simulink model "Simulink_AM"  (R2020b)
settings: Solver=VariableStepAuto  StartTime=0.0  StopTime=10.0  RelTol=1e-3
libraries: dsparch4 x2
settings Model: Creator=enrique  LastModifiedBy=enrique

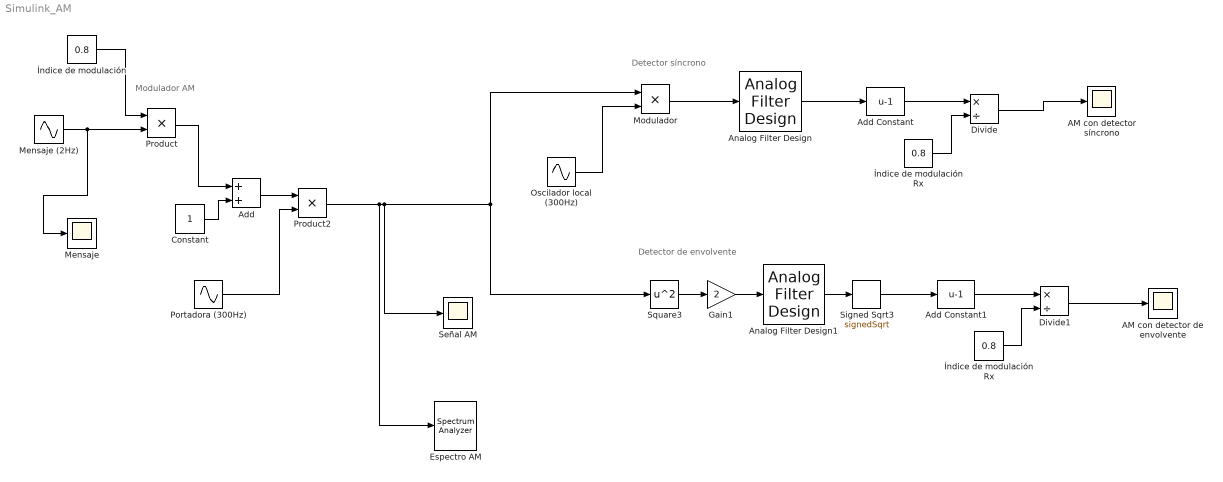
== system Simulink_AM ==
  note: Detector de envolvente
  note: Detector síncrono
  note: Modulador AM
  AM con detector de envolvente : Scope
  AM con detector síncrono : Scope
  Add : Sum
  Add Constant : Bias  Bias=-1
  Add Constant1 : Bias  Bias=-1
  Analog Filter Design : dsparch4/Analog Filter Design  method=Butterworth  filttype=Lowpass  N=4  Wlo=2*pi*5  Whi=80  Rp=2  Rs=40
  Analog Filter Design1 : dsparch4/Analog Filter Design  method=Butterworth  filttype=Lowpass  N=4  Wlo=2*pi*10  Whi=80  Rp=2  Rs=40
  Constant : Constant
  Divide : Product  Inputs=*/
  Divide1 : Product  Inputs=*/
  Espectro AM : SpectrumAnalyzer
  Gain1 : Gain  Gain=2
  Mensaje : Scope
  "Mensaje (2Hz) " : Sin  Frequency=2*pi*2  SampleTime=1/5000
  Modulador : Product  OutDataTypeStr=Inherit: Same as first input
  Oscilador local (300Hz) : Sin  Amplitude=2  Frequency=2*pi*300  SampleTime=1/5000
  "Portadora (300Hz) " : Sin  Frequency=2*pi*300  SampleTime=1/5000
  Product : Product
  Product2 : Product  OutDataTypeStr=Inherit: Same as first input
  Señal AM : Scope
  Signed Sqrt3 : Sqrt  Operator=signedSqrt  SaturateOnIntegerOverflow=on
  Square3 : Math  Operator=square  SaturateOnIntegerOverflow=on
  Índice de modulación : Constant  Value=0.8
  Índice de modulación Rx : Constant  Value=0.8
  "Índice de modulación Rx " : Constant  Value=0.8
  wires:
  Índice de modulación/1 -> Product/1
  Constant/1 -> Add/2
  Add/1 -> Product2/1
  Product/1 -> Add/1
  "Portadora (300Hz) "/1 -> Product2/2
  "Mensaje (2Hz) "/1 -> Product/2, Mensaje/1
  Oscilador local (300Hz)/1 -> Modulador/2
  Modulador/1 -> Analog Filter Design/1
  Analog Filter Design1/1 -> Signed Sqrt3/1
  Square3/1 -> Gain1/1
  Gain1/1 -> Analog Filter Design1/1
  Product2/1 -> Square3/1, Modulador/1, Señal AM/1, Espectro AM/1
  Analog Filter Design/1 -> Add Constant/1
  Divide/1 -> AM con detector síncrono/1
  Add Constant/1 -> Divide/1
  Índice de modulación Rx/1 -> Divide/2
  Add Constant1/1 -> Divide1/1
  "Índice de modulación Rx "/1 -> Divide1/2
  Signed Sqrt3/1 -> Add Constant1/1
  Divide1/1 -> AM con detector de envolvente/1
